simulink model "NoAxleCompliances"  (R2026b)
settings: Solver=VariableStepAuto
settings Model: ModifiedByFormat=The MathWorks, Inc.  Creator=The MathWorks, Inc.  LastModifiedBy=The MathWorks, Inc.

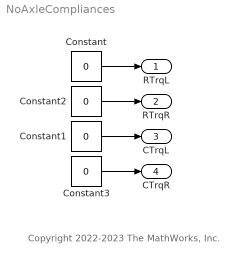
== system NoAxleCompliances ==
  note: Copyright 2022-2023 The MathWorks, Inc.
  Constant{,1..3} (4 alike) : Constant  Value=0  SampleTime=-1
  RTrqL : Outport
  RTrqR : Outport  Port=2
  CTrqL : Outport  Port=3
  CTrqR : Outport  Port=4
  wires:
  Constant2/1 -> RTrqR/1
  Constant1/1 -> CTrqL/1
  Constant/1 -> RTrqL/1
  Constant3/1 -> CTrqR/1
